simulink model "Practica"  (R2021a)
settings: Solver=VariableStepAuto  StartTime=0.0  StopTime=10.0  RelTol=1e-3
undefined symbols (not defined in the file): b1, b2
libraries: dspsnks4 x1, dspvision x1
settings Model: Creator=jheym  LastModifiedBy=jheym

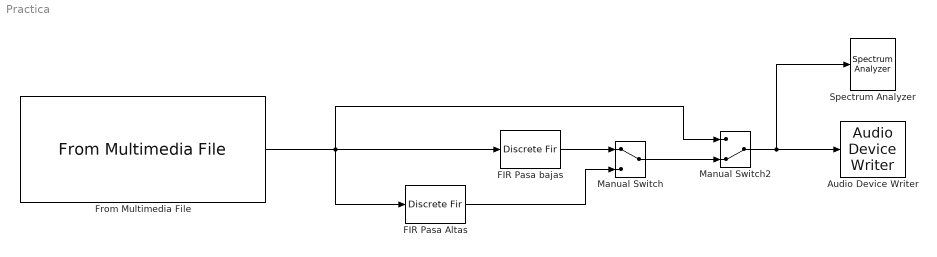
== system Practica ==
  Audio Device Writer : dspsnks4/Audio Device Writer  Driver=DirectSound  Device=Default  InheritSampleRate=on  SampleRate=44100  BitDepth=16-bit integer  BufferSize=4096  NumBuffers=10  DefaultOutputChannelMapping=on  OutputChannelMapping=1:2  OutputNumUnderrunSamples=off  DriverIdx=1  DeviceWarnFlag=''
  FIR Pasa Altas : DiscreteFir  Coefficients=b2
  FIR Pasa bajas : DiscreteFir  Coefficients=b1
  From Multimedia File : dspvision/From Multimedia File  inputFilename=E:\Documentos\Laboral\UPIEM\Procesamiento de señales digitales\traimory-mega-horn-angry-siren-f-cinematic-trailer-sound-effects-193408.mp3  readRange=[1 Inf]  loop=on  numPlays=inf  outputStreams=Audio only  videoDataType=single  audioDataType=double  inheritSampleTime=on  userDefinedSampleTime=1/30  noAudioOutput=off  isIntensityVideo=off  fourcc=RGB  colorVideoFormat=Separate color signals  outputEOF=off  dataOrg=Column-major  audioFrameSize=1024  computeAudioFrameSize=off  outSamplingMode=Sample based
  Manual Switch : ManualSwitch
  Manual Switch2 : ManualSwitch  CurrentSetting=0
  Spectrum Analyzer : SpectrumAnalyzer
  wires:
  FIR Pasa bajas/1 -> Manual Switch/1
  FIR Pasa Altas/1 -> Manual Switch/2
  From Multimedia File/1 -> Manual Switch2/1, FIR Pasa Altas/1, FIR Pasa bajas/1
  Manual Switch/1 -> Manual Switch2/2
  Manual Switch2/1 -> Spectrum Analyzer/1, Audio Device Writer/1
